simulink model "ssc_pd"  (R2014a)
settings: Solver=ode45  StartTime=0.0  StopTime=10.0  RelTol=1e-3
undefined symbols (not defined in the file or in its folder): q, qd, qdd
settings Model: Creator=user  LastModifiedBy=Wolfgang
settings SolverCC: ZeroCrossAlgorithm=Adaptive
settings OptimizationCC: SimCompilerOptimization=On
settings DebuggingCC: UnderspecifiedInitializationDetection=Classic  SolverPrmCheckMsg=none

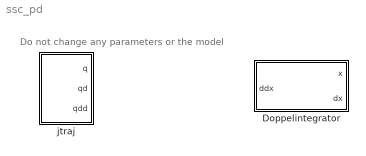
== system ssc_pd ==
  note: Do not change any parameters or the model
  Doppelintegrator : Subsystem
      mask Display: dpoly([1],[1 0 0], 's')
  jtraj : Subsystem  mask{q0=0, qf=pi/2, tmax=10}
      mask help: Joint interpolated trajectory.
      mask init:
      | n = length(q0);
      | if length(q0) ~= length(qf) ,
      |  error('q0 and qf must be same length')
      | end
      | t=[0:100]'/100*tmax;
      | [q,qd,qdd] = jtraj(q0, qf, t);
      mask Help:
      | Generate quintic polynomial to move from initial to final joint angles as specified.  Initial and final velocity are assumed to be zero.
      | 
      | Outputs joint angles as well as joint angle rates.
      mask Display:
      | port_label('output', 1, 'q')
      | port_label('output', 2, 'qd')
      | port_label('output', 3, 'qdd')

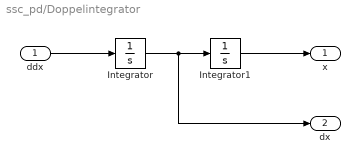
== system ssc_pd/Doppelintegrator ==
  ddx : Inport
  Integrator : Integrator
  Integrator1 : Integrator
  x : Outport
  dx : Outport  Port=2
  wires:
  Integrator/1 -> dx/1, Integrator1/1
  Integrator1/1 -> x/1
  ddx/1 -> Integrator/1

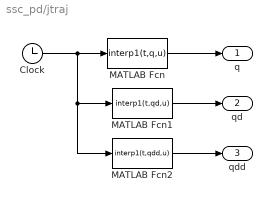
== system ssc_pd/jtraj ==
  Clock : Clock
  MATLAB Fcn : MATLABFcn  MATLABFcn=interp1(t,q,u)  OutputDimensions=n
  MATLAB Fcn1 : MATLABFcn  MATLABFcn=interp1(t,qd,u)  OutputDimensions=n
  MATLAB Fcn2 : MATLABFcn  MATLABFcn=interp1(t,qdd,u)  OutputDimensions=n
  q : Outport
  qd : Outport  Port=2
  qdd : Outport  Port=3
  wires:
  MATLAB Fcn2/1 -> qdd/1
  Clock/1 -> MATLAB Fcn2/1, MATLAB Fcn1/1, MATLAB Fcn/1
  MATLAB Fcn1/1 -> qd/1
  MATLAB Fcn/1 -> q/1
